simulink model "ADC_reader_simulink"  (R2025a)
settings: Solver=FixedStepAuto  StartTime=0.0  StopTime=inf  FixedStep=0.01  RelTol=1e-3  EnableMultiTasking=on
libraries: stm32f4xxblockslib x7
settings Model: STM32="{\"AnalogInput\":[{\"ID\":\"test_poten:20\"},{\"ID\":\"test_poten:28\"},{\"ID\":\"ADC_reader:28\"},{\"ID\":\"ADC_reader:20\"},{\"ID\":\"ADC_reader:14\"},{\"ID\":\"ADC_reader:11\"},{\"ID\":\"ADC_reader:8\"},{\"ID\":\"ADC_reader:5\"},{\"ID\":\"ADC_reader:1\"},{\"ID\":\"ADC_reader_simulink:14\"},{\"ID\":\"ADC_reader_simulink:11\"},{\"ID\":\"ADC_reader_simulink:8\"},{\"ID\":\"ADC_reader_simulink:5\"},{\"ID\":\"ADC_reader_simulink:1\"},{\"ID\":\"ADC_reader_simulink:20\"}]}"  Creator=ioonz  LastModifiedBy=nitic
settings OptimizationCC: DefaultParameterBehavior=Inlined  EnhancedBackFolding=on  PassReuseOutputArgsAs=Individual arguments  ZeroExternalMemoryAtStartup=off  ZeroInternalMemoryAtStartup=off  MaxStackSize=512  OptimizeBlockOrder=speed  DifferentSizesBufferReuse=on  OptimizationCustomize=off  EfficientTunableParamExpr=on
settings DebuggingCC: ParameterTunabilityLossMsg=error
settings HardwareCC: ProdBitPerPointer=32.0  ProdBitPerSizeT=32.0  ProdBitPerPtrDiffT=32.0  ProdLargestAtomicInteger=Long  ProdLargestAtomicFloat=Double  ProdWordSize=32.0  ProdLongLongMode=on  ProdHWDeviceType=ARM Compatible->ARM Cortex-M
settings SFSimCC: MATLABDynamicMemAlloc=off
settings RTWCC: SystemTargetFile=ert.tlc  HardwareBoard=STM32G4xx Based  TemplateMakefile=ert_default_tmf  Toolchain=GNU Tools for ARM Embedded Processors  Description=Embedded Coder
settings CodeAppCC: ForceParamTrailComments=on  IgnoreCustomStorageClasses=off  OperatorAnnotations=on  SimulinkDataObjDesc=on  SFDataObjDesc=on  InsertBlockDesc=on
settings ERTTargetCC: ExtModeTransport=3.0  ExtModeStaticAllocSize=2048.0  TargetLangStandard=C99 (ISO)  CodeReplacementLibrary=ARM Cortex-M

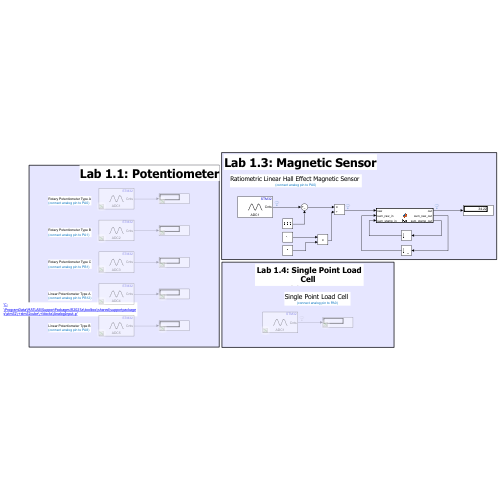
[thumbnail: Simulink's stored preview of the top-level diagram]
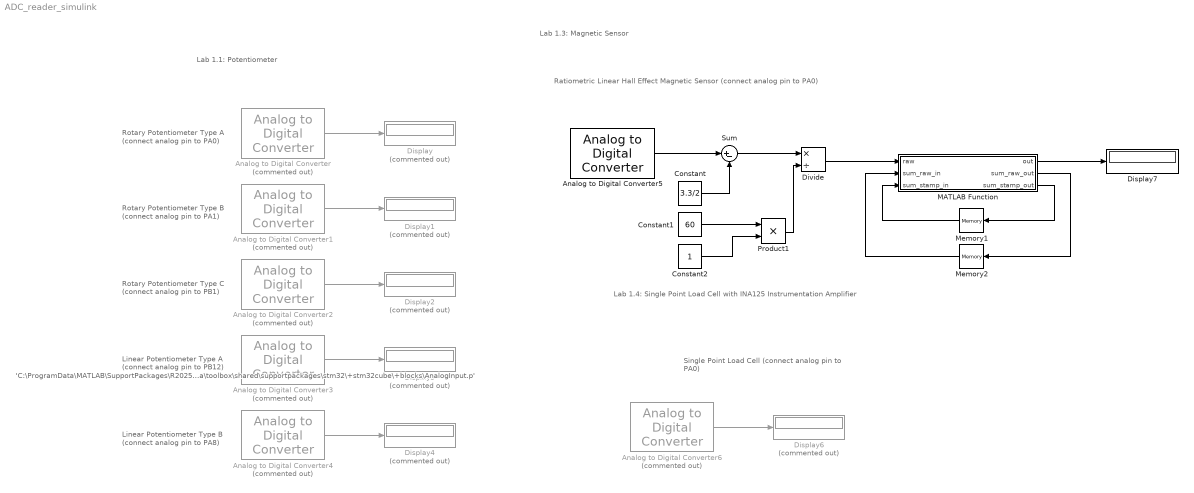
== system ADC_reader_simulink ==
  note: 'C:\ProgramData\MATLAB\SupportPackages\R2025a\toolbox\shared\supportpackages\stm32\+stm32cube\+blocks\AnalogInput.p'
  note: Lab 1.1: Potentiometer
  note: Rotary Potentiometer Type A
      | (connect analog pin to PA0)
  note: Rotary Potentiometer Type B
      | (connect analog pin to PA1)
  note: Rotary Potentiometer Type C
      | (connect analog pin to PB1)
  note: Linear Potentiometer Type A
      | (connect analog pin to PB12)
  note: Linear Potentiometer Type B
      | (connect analog pin to PA8)
  note: Ratiometric Linear Hall Effect Magnetic Sensor
      | (connect analog pin to PA0)
  note: Single Point Load Cell
      | (connect analog pin to PA0)
  note: Lab 1.3: Magnetic Sensor
  note: Lab 1.4: Single Point Load Cell
      | with INA125 Instrumentation Amplifier
  Analog to Digital Converter : stm32f4xxblockslib/Analog to Digital Converter  Commented=on  ADCModule=ADC1  ConversionGroup=Regular  TriggerMode=Trigger and read  NumberOfConversions=1  EnableBufferConv=off  BufferLength=1  OutputStatus=off  SampleTime=-1  EnableSimPort=off  hoistedMaskSrc=ECSoC/ECSimCodegen/Analog to Digital Converter
  Analog to Digital Converter1 : stm32f4xxblockslib/Analog to Digital Converter  Commented=on  ADCModule=ADC2  ConversionGroup=Regular  TriggerMode=Trigger and read  NumberOfConversions=1  EnableBufferConv=off  BufferLength=1  OutputStatus=off  SampleTime=-1  EnableSimPort=off  hoistedMaskSrc=ECSoC/ECSimCodegen/Analog to Digital Converter
  Analog to Digital Converter2 : stm32f4xxblockslib/Analog to Digital Converter  Commented=on  ADCModule=ADC3  ConversionGroup=Regular  TriggerMode=Trigger and read  NumberOfConversions=1  EnableBufferConv=off  BufferLength=1  OutputStatus=off  SampleTime=-1  EnableSimPort=off  hoistedMaskSrc=ECSoC/ECSimCodegen/Analog to Digital Converter
  Analog to Digital Converter3 : stm32f4xxblockslib/Analog to Digital Converter  Commented=on  ADCModule=ADC4  ConversionGroup=Regular  TriggerMode=Trigger and read  NumberOfConversions=1  EnableBufferConv=off  BufferLength=1  OutputStatus=off  SampleTime=-1  EnableSimPort=off  hoistedMaskSrc=ECSoC/ECSimCodegen/Analog to Digital Converter
  Analog to Digital Converter4 : stm32f4xxblockslib/Analog to Digital Converter  Commented=on  ADCModule=ADC5  ConversionGroup=Regular  TriggerMode=Trigger and read  NumberOfConversions=1  EnableBufferConv=off  BufferLength=1  OutputStatus=off  SampleTime=-1  EnableSimPort=off  hoistedMaskSrc=ECSoC/ECSimCodegen/Analog to Digital Converter
  Analog to Digital Converter5 : stm32f4xxblockslib/Analog to Digital Converter  ADCModule=ADC1  ConversionGroup=Regular  TriggerMode=Trigger and read  NumberOfConversions=1  EnableBufferConv=off  BufferLength=1  OutputStatus=off  SampleTime=-1  EnableSimPort=off  hoistedMaskSrc=ECSoC/ECSimCodegen/Analog to Digital Converter
  Analog to Digital Converter6 : stm32f4xxblockslib/Analog to Digital Converter  Commented=on  ADCModule=ADC1  ConversionGroup=Regular  TriggerMode=Trigger and read  NumberOfConversions=1  EnableBufferConv=off  BufferLength=1  OutputStatus=off  SampleTime=-1  EnableSimPort=off  hoistedMaskSrc=ECSoC/ECSimCodegen/Analog to Digital Converter
  Constant : Constant  Value=3.3/2
  Constant1 : Constant  Value=60
  Constant2 : Constant
  Display{,1..4,6} (6 alike) : Display  Commented=on
  Display7 : Display
  Divide : Product  Inputs=*/
  MATLAB Function : MATLAB Function  TreatAsAtomicUnit=on
  Memory1 : Memory
  Memory2 : Memory
  Product1 : Product
  Sum : Sum  Inputs=|+-
  wires:
  Analog to Digital Converter/1 -> Display/1
  Analog to Digital Converter1/1 -> Display1/1
  Analog to Digital Converter2/1 -> Display2/1
  Analog to Digital Converter3/1 -> Display3/1
  Analog to Digital Converter4/1 -> Display4/1
  Analog to Digital Converter5/1 -> Sum/1
  Analog to Digital Converter6/1 -> Display6/1
  Constant/1 -> Sum/2
  Sum/1 -> Divide/1
  Constant1/1 -> Product1/1
  Constant2/1 -> Product1/2
  Product1/1 -> Divide/2
  MATLAB Function/1(out) -> Display7/1
  MATLAB Function/3(sum_stamp_out) -> Memory1/1
  Memory1/1 -> MATLAB Function/3(sum_stamp_in)
  MATLAB Function/2(sum_raw_out) -> Memory2/1
  Memory2/1 -> MATLAB Function/2(sum_raw_in)
  Divide/1 -> MATLAB Function/1(raw)

== matlab function ADC_reader_simulink/MATLAB Function ==
  data: raw input; sum_raw_in input; out output; sum_stamp_in input; sum_raw_out output; sum_stamp_out output
function [out,sum_raw_out,sum_stamp_out] = fcn(raw, sum_raw_in, sum_stamp_in)

if sum_stamp_in == 100
    sum_stamp_out = sum_stamp_in + 1;
    sum_raw_out =  sum_raw_in + raw;
    out = (sum_raw_out)/(sum_stamp_out);
    sum_stamp_out = 0;
    sum_raw_out = 0;
else
    sum_stamp_out = sum_stamp_in + 1;
    sum_raw_out =  sum_raw_in + raw;
    out = (sum_raw_out)/(sum_stamp_out);
end
